simulink model "inverter_spwm_sixty_phases"  (R2024b)
settings: Solver=VariableStepAuto  StartTime=0.0  StopTime=0.1  RelTol=1e-3
libraries: spsMosfetLib x132, spsSeriesRLCBranchLib x65, spsCurrentMeasurementLib x64, spsVoltageMeasurementLib x64, spsTriangleGeneratorLib x20, spsDCVoltageSourceLib x4, spsGroundLib x2, spsThreePhaseSeriesRLCBranchLib x1, sps_lib x1
(part 1 of 2)
settings Model: Creator=Harry  LastModifiedBy=Harry

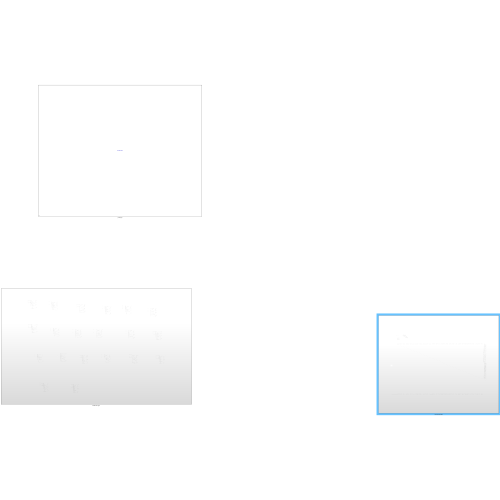
[thumbnail: Simulink's stored preview of the top-level diagram]
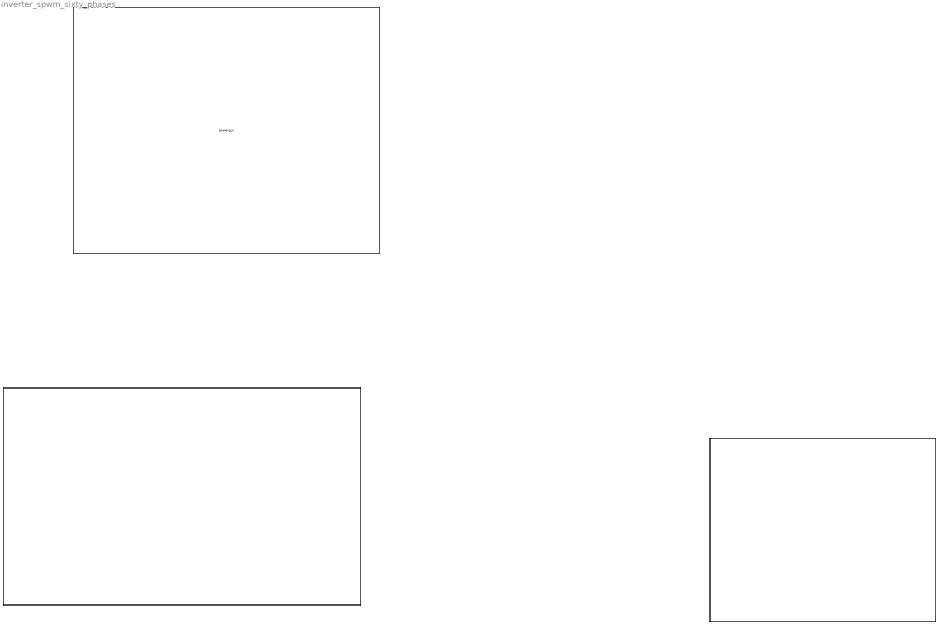
== system inverter_spwm_sixty_phases ==
  Dead time logic : Subsystem
  Inverter switches : Subsystem
  powergui : sps_lib/powergui  Priority=1  SimulationMode=Continuous  SampleTime=50e-6  frequency=60  Iterations=50  frequencyindice=0  Pbase=100e6  ErrMax=1e-4  UnitsV=kV  UnitsW=MW  buscounter=0  FunctionMessages=off  echomessages=off  EnableUseOfTLC=off  CurrentSourceSwitches=off  DisableSnubberDevices=off  DisableRonSwitches=off  DisableVfSwitches=off  DisplayEquations=off  AutomaticDiscreteSolvers=off  SolverType=Tustin/Backward Euler (TBE)  Interpol=off  ExternalGateDelay=off  methode=off  Ts=100  x0status=blocks  SPID=on  SwTol=0  HookPort=off  NonlinearTolerance=1e-4  nMaxIteration=100  ContinueOnMaxIteration=off  RestoreLinks=warning  ResistiveCurrentMeasurement=off  Frange=[0:2:500]  Ylog=off  Xlog=on  ShowGrid=off  save=off  variable=ZData  structure=0  ZoomFFT=off  StartTime=0.0  cycles=1  DisplayStyle=1  fundamental=60  FreqAxis=off  MaxFrequency=1000  frequencyindicesteady=1  RmsSteady=1  display=off

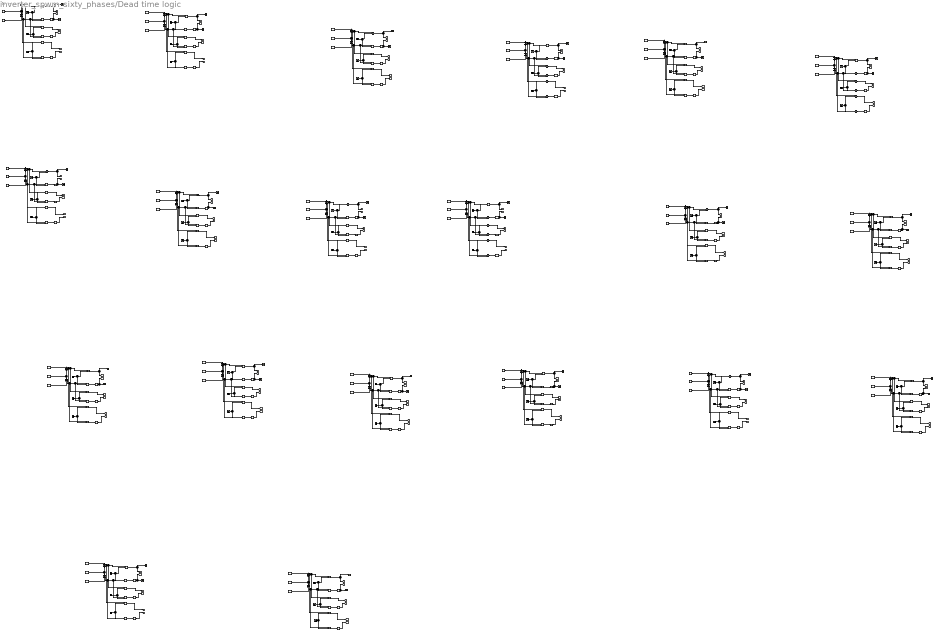
== system inverter_spwm_sixty_phases/Dead time logic ==
  Add{1,3,5,7,9,11,13,15,17,19,21,23,25,27,29,31,33,35,37,39} (20 alike) : Sum
  Add{2,4,6,8,10,12,14,16,18,20,22,24,26,28,30,32,34,36,38,40} (20 alike) : Sum  Inputs=+-
  Constant{1..40} (40 alike) : Constant  Value=0.1
  NOT{1..60} (60 alike) : Logic  Operator=NOT  AllPortsSameDT=off  OutDataTypeStr=boolean
  Relational Operator{,1..119} (120 alike) : RelationalOperator  Operator=<=  OutDataTypeStr=boolean  RndMeth=Simplest  InputSameDT=off
  Scope{,1..39} (40 alike) : Scope
  Sine Wave1 : Sin  Amplitude=0.961  Frequency=2*pi*25  Phase=18*pi/180  SampleTime=0
  Sine Wave10 : Sin  Amplitude=0.961  Frequency=2*pi*25  Phase=54*pi/180  SampleTime=0
  Sine Wave11 : Sin  Amplitude=0.961  Frequency=2*pi*25  Phase=60*pi/180  SampleTime=0
  Sine Wave12 : Sin  Amplitude=0.961  Frequency=2*pi*25  Phase=66*pi/180  SampleTime=0
  Sine Wave13 : Sin  Amplitude=0.961  Frequency=2*pi*25  Phase=72*pi/180  SampleTime=0
  Sine Wave14 : Sin  Amplitude=0.961  Frequency=2*pi*25  Phase=78*pi/180  SampleTime=0
  Sine Wave15 : Sin  Amplitude=0.961  Frequency=2*pi*25  Phase=84*pi/180  SampleTime=0
  Sine Wave16 : Sin  Amplitude=0.961  Frequency=2*pi*25  Phase=90*pi/180  SampleTime=0
  Sine Wave17 : Sin  Amplitude=0.961  Frequency=2*pi*25  Phase=96*pi/180  SampleTime=0
  Sine Wave18 : Sin  Amplitude=0.961  Frequency=2*pi*25  Phase=102*pi/180  SampleTime=0
  Sine Wave19 : Sin  Amplitude=0.961  Frequency=2*pi*25  Phase=324*pi/180  SampleTime=0
  Sine Wave2 : Sin  Amplitude=0.961  Frequency=2*pi*25  Phase=24*pi/180  SampleTime=0
  Sine Wave20 : Sin  Amplitude=0.961  Frequency=2*pi*25  Phase=330*pi/180  SampleTime=0
  Sine Wave21 : Sin  Amplitude=0.961  Frequency=2*pi*25  Phase=336*pi/180  SampleTime=0
  Sine Wave22 : Sin  Amplitude=0.961  Frequency=2*pi*25  Phase=108*pi/180  SampleTime=0
  Sine Wave23 : Sin  Amplitude=0.961  Frequency=2*pi*25  Phase=114*pi/180  SampleTime=0
  Sine Wave24 : Sin  Amplitude=0.961  Frequency=2*pi*25  Phase=120*pi/180  SampleTime=0
  Sine Wave25 : Sin  Amplitude=0.961  Frequency=2*pi*25  Phase=126*pi/180  SampleTime=0
  Sine Wave26 : Sin  Amplitude=0.961  Frequency=2*pi*25  Phase=132*pi/180  SampleTime=0
  Sine Wave27 : Sin  Amplitude=0.961  Frequency=2*pi*25  Phase=138*pi/180  SampleTime=0
  Sine Wave28 : Sin  Amplitude=0.961  Frequency=2*pi*25  Phase=144*pi/180  SampleTime=0
  Sine Wave29 : Sin  Amplitude=0.961  Frequency=2*pi*25  Phase=150*pi/180  SampleTime=0
  Sine Wave3 : Sin  Amplitude=0.961  Frequency=2*pi*25  Phase=30*pi/180  SampleTime=0
  Sine Wave30 : Sin  Amplitude=0.961  Frequency=2*pi*25  Phase=156*pi/180  SampleTime=0
  Sine Wave31 : Sin  Amplitude=0.961  Frequency=2*pi*25  Phase=162*pi/180  SampleTime=0
  Sine Wave32 : Sin  Amplitude=0.961  Frequency=2*pi*25  Phase=168*pi/180  SampleTime=0
  Sine Wave33 : Sin  Amplitude=0.961  Frequency=2*pi*25  Phase=174*pi/180  SampleTime=0
  Sine Wave34 : Sin  Amplitude=0.961  Frequency=2*pi*25  Phase=180*pi/180  SampleTime=0
  Sine Wave35 : Sin  Amplitude=0.961  Frequency=2*pi*25  Phase=186*pi/180  SampleTime=0
  Sine Wave36 : Sin  Amplitude=0.961  Frequency=2*pi*25  Phase=192*pi/180  SampleTime=0
  Sine Wave37 : Sin  Amplitude=0.961  Frequency=2*pi*25  Phase=198*pi/180  SampleTime=0
  Sine Wave38 : Sin  Amplitude=0.961  Frequency=2*pi*25  Phase=204*pi/180  SampleTime=0
  Sine Wave39 : Sin  Amplitude=0.961  Frequency=2*pi*25  Phase=210*pi/180  SampleTime=0
  Sine Wave4 : Sin  Amplitude=0.961  Frequency=2*pi*25  SampleTime=0
  Sine Wave40 : Sin  Amplitude=0.961  Frequency=2*pi*25  Phase=216*pi/180  SampleTime=0
  Sine Wave41 : Sin  Amplitude=0.961  Frequency=2*pi*25  Phase=222*pi/180  SampleTime=0
  Sine Wave42 : Sin  Amplitude=0.961  Frequency=2*pi*25  Phase=228*pi/180  SampleTime=0
  Sine Wave43 : Sin  Amplitude=0.961  Frequency=2*pi*25  Phase=234*pi/180  SampleTime=0
  Sine Wave44 : Sin  Amplitude=0.961  Frequency=2*pi*25  Phase=240*pi/180  SampleTime=0
  Sine Wave45 : Sin  Amplitude=0.961  Frequency=2*pi*25  Phase=246*pi/180  SampleTime=0
  Sine Wave46 : Sin  Amplitude=0.961  Frequency=2*pi*25  Phase=252*pi/180  SampleTime=0
  Sine Wave47 : Sin  Amplitude=0.961  Frequency=2*pi*25  Phase=258*pi/180  SampleTime=0
  Sine Wave48 : Sin  Amplitude=0.961  Frequency=2*pi*25  Phase=264*pi/180  SampleTime=0
  Sine Wave49 : Sin  Amplitude=0.961  Frequency=2*pi*25  Phase=270*pi/180  SampleTime=0
  Sine Wave5 : Sin  Amplitude=0.961  Frequency=2*pi*25  Phase=6*pi/180  SampleTime=0
  Sine Wave50 : Sin  Amplitude=0.961  Frequency=2*pi*25  Phase=276*pi/180  SampleTime=0
  Sine Wave51 : Sin  Amplitude=0.961  Frequency=2*pi*25  Phase=282*pi/180  SampleTime=0
  Sine Wave52 : Sin  Amplitude=0.961  Frequency=2*pi*25  Phase=288*pi/180  SampleTime=0
  Sine Wave53 : Sin  Amplitude=0.961  Frequency=2*pi*25  Phase=294*pi/180  SampleTime=0
  Sine Wave54 : Sin  Amplitude=0.961  Frequency=2*pi*25  Phase=300*pi/180  SampleTime=0
  Sine Wave55 : Sin  Amplitude=0.961  Frequency=2*pi*25  Phase=306*pi/180  SampleTime=0
  Sine Wave56 : Sin  Amplitude=0.961  Frequency=2*pi*25  Phase=312*pi/180  SampleTime=0
  Sine Wave57 : Sin  Amplitude=0.961  Frequency=2*pi*25  Phase=318*pi/180  SampleTime=0
  Sine Wave58 : Sin  Amplitude=0.961  Frequency=2*pi*25  Phase=342*pi/180  SampleTime=0
  Sine Wave59 : Sin  Amplitude=0.961  Frequency=2*pi*25  Phase=348*pi/180  SampleTime=0
  Sine Wave6 : Sin  Amplitude=0.961  Frequency=2*pi*25  Phase=12*pi/180  SampleTime=0
  Sine Wave60 : Sin  Amplitude=0.961  Frequency=2*pi*25  Phase=354*pi/180  SampleTime=0
  Sine Wave7 : Sin  Amplitude=0.961  Frequency=2*pi*25  Phase=36*pi/180  SampleTime=0
  Sine Wave8 : Sin  Amplitude=0.961  Frequency=2*pi*25  Phase=42*pi/180  SampleTime=0
  Sine Wave9 : Sin  Amplitude=0.961  Frequency=2*pi*25  Phase=48*pi/180  SampleTime=0
  Triangle Generator{,1..19} (20 alike) : spsTriangleGeneratorLib/Triangle Generator  Freq=2000  Phase=90  Ts=0
  tag scope: s100=global, s101=global, s102=global, s103=global, s104=global, s105=global, s106=global, s107=global, s108=global, s109=global, s10=global, s110=global, s111=global, s112=global, s113=global, s114=global, s115=global, s116=global, s117=global, s118=global, s119=global, s11=global, s120=global, s12=global, s13=global, s14=global, s15=global, s16=global, s17=global, s18=global, s19=global, s1=global, s20=global, s21=global, s22=global, s23=global, s24=global, s25=global, s26=global, s27=global, s28=global, s29=global, s2=global, s30=global, s31=global, s32=global, s33=global, s34=global, s35=global, s36=global, s37=global, s38=global, s39=global, s3=global, s40=global, s41=global, s42=global, s43=global, s44=global, s45=global, s46=global, s47=global, s48=global, s49=global, s4=global, s50=global, s51=global, s52=global, s53=global, s54=global, s55=global, s56=global, s57=global, s58=global, s59=global, s5=global, s60=global, s61=global, s62=global, s63=global, s64=global, s65=global, s66=global, s67=global, s68=global, s69=global, s6=global, s70=global, s71=global, s72=global, s73=global, s74=global, s75=global, s76=global, s77=global, s78=global, s79=global, s7=global, s80=global, s81=global, s82=global, s83=global, s84=global, s85=global, s86=global, s87=global, s88=global, s89=global, s8=global, s90=global, s91=global, s92=global, s93=global, s94=global, s95=global, s96=global, s97=global, s98=global, s99=global, s9=global
  wires:
  Relational Operator5/1 -> NOT5/1
  Add8/1 -> Relational Operator4/1, Relational Operator5/1, Relational Operator1/1
  Relational Operator3/1 -> [s5]
  Sine Wave4/1 -> Relational Operator/2, Relational Operator1/2
  Sine Wave6/1 -> Relational Operator4/2, Relational Operator3/2
  Relational Operator2/1 -> [s3]
  Sine Wave5/1 -> Relational Operator5/2, Relational Operator2/2
  Relational Operator4/1 -> NOT6/1
  Triangle Generator/1 -> Add8/1, Add7/2
  NOT5/1 -> [s4]
  Relational Operator1/1 -> NOT4/1
  NOT6/1 -> [s6]
  Constant2/1 -> Add7/1
  Relational Operator/1 -> [s1], Scope1/1
  Constant3/1 -> Add8/2
  NOT4/1 -> [s2], Scope/1
  Add7/1 -> Relational Operator3/1, Relational Operator2/1, Relational Operator/1
  NOT24/1 -> [s42]
  Triangle Generator7/1 -> Add16/1, Add15/2
  Sine Wave23/1 -> Relational Operator47/2, Relational Operator44/2
  Sine Wave22/1 -> Relational Operator42/2, Relational Operator43/2
  Relational Operator44/1 -> [s39]
  Relational Operator43/1 -> NOT22/1
  Sine Wave24/1 -> Relational Operator46/2, Relational Operator45/2
  Relational Operator45/1 -> [s41]
  Relational Operator47/1 -> NOT23/1
  Add16/1 -> Relational Operator46/1, Relational Operator47/1, Relational Operator43/1
  Relational Operator46/1 -> NOT24/1
  Constant16/1 -> Add16/2
  NOT22/1 -> [s38], Scope14/1
  Relational Operator42/1 -> [s37], Scope15/1
  Constant15/1 -> Add15/1
  Add15/1 -> Relational Operator45/1, Relational Operator44/1, Relational Operator42/1
  NOT23/1 -> [s40]
  NOT27/1 -> [s48]
  Triangle Generator8/1 -> Add18/1, Add17/2
  Sine Wave26/1 -> Relational Operator53/2, Relational Operator50/2
  Sine Wave25/1 -> Relational Operator48/2, Relational Operator49/2
  Relational Operator50/1 -> [s45]
  Relational Operator49/1 -> NOT25/1
  Sine Wave27/1 -> Relational Operator52/2, Relational Operator51/2
  Relational Operator51/1 -> [s47]
  Relational Operator53/1 -> NOT26/1
  Add18/1 -> Relational Operator52/1, Relational Operator53/1, Relational Operator49/1
  Relational Operator52/1 -> NOT27/1
  Constant18/1 -> Add18/2
  NOT25/1 -> [s44], Scope16/1
  Relational Operator48/1 -> [s43], Scope17/1
  Constant17/1 -> Add17/1
  Add17/1 -> Relational Operator51/1, Relational Operator50/1, Relational Operator48/1
  NOT26/1 -> [s46]
  NOT30/1 -> [s54]
  Triangle Generator9/1 -> Add20/1, Add19/2
  Sine Wave29/1 -> Relational Operator59/2, Relational Operator56/2
  Sine Wave28/1 -> Relational Operator54/2, Relational Operator55/2
  Relational Operator56/1 -> [s51]
  Relational Operator55/1 -> NOT28/1
  Sine Wave30/1 -> Relational Operator58/2, Relational Operator57/2
  Relational Operator57/1 -> [s53]
  Relational Operator59/1 -> NOT29/1
  Add20/1 -> Relational Operator58/1, Relational Operator59/1, Relational Operator55/1
  Relational Operator58/1 -> NOT30/1
  Constant20/1 -> Add20/2
  NOT28/1 -> [s50], Scope18/1
  Relational Operator54/1 -> [s49], Scope19/1
  Constant19/1 -> Add19/1
  Add19/1 -> Relational Operator57/1, Relational Operator56/1, Relational Operator54/1
  NOT29/1 -> [s52]
  NOT33/1 -> [s60]
  Triangle Generator10/1 -> Add22/1, Add21/2
  Sine Wave32/1 -> Relational Operator65/2, Relational Operator62/2
  Sine Wave31/1 -> Relational Operator60/2, Relational Operator61/2
  Relational Operator62/1 -> [s57]
  Relational Operator61/1 -> NOT31/1
  Sine Wave33/1 -> Relational Operator64/2, Relational Operator63/2
  Relational Operator63/1 -> [s59]
  Relational Operator65/1 -> NOT32/1
  Add22/1 -> Relational Operator64/1, Relational Operator65/1, Relational Operator61/1
  Relational Operator64/1 -> NOT33/1
  Constant22/1 -> Add22/2
  NOT31/1 -> [s56], Scope20/1
  Relational Operator60/1 -> [s55], Scope21/1
  Constant21/1 -> Add21/1
  Add21/1 -> Relational Operator63/1, Relational Operator62/1, Relational Operator60/1
  NOT32/1 -> [s58]
  NOT36/1 -> [s66]
  Triangle Generator11/1 -> Add24/1, Add23/2
  Sine Wave35/1 -> Relational Operator71/2, Relational Operator68/2
  Sine Wave34/1 -> Relational Operator66/2, Relational Operator67/2
  Relational Operator68/1 -> [s63]
  Relational Operator67/1 -> NOT34/1
  Sine Wave36/1 -> Relational Operator70/2, Relational Operator69/2
  Relational Operator69/1 -> [s65]
  Relational Operator71/1 -> NOT35/1
  Add24/1 -> Relational Operator70/1, Relational Operator71/1, Relational Operator67/1
  Relational Operator70/1 -> NOT36/1
  Constant24/1 -> Add24/2
  NOT34/1 -> [s62], Scope22/1
  Relational Operator66/1 -> [s61], Scope23/1
  Constant23/1 -> Add23/1
  Add23/1 -> Relational Operator69/1, Relational Operator68/1, Relational Operator66/1
  NOT35/1 -> [s64]
  NOT39/1 -> [s72]
  Triangle Generator12/1 -> Add26/1, Add25/2
  Sine Wave38/1 -> Relational Operator77/2, Relational Operator74/2
  Sine Wave37/1 -> Relational Operator72/2, Relational Operator73/2
  Relational Operator74/1 -> [s69]
  Relational Operator73/1 -> NOT37/1
  Sine Wave39/1 -> Relational Operator76/2, Relational Operator75/2
  Relational Operator75/1 -> [s71]
  Relational Operator77/1 -> NOT38/1
  Add26/1 -> Relational Operator76/1, Relational Operator77/1, Relational Operator73/1
  Relational Operator76/1 -> NOT39/1
  Constant26/1 -> Add26/2
  NOT37/1 -> [s68], Scope24/1
  Relational Operator72/1 -> [s67], Scope25/1
  Constant25/1 -> Add25/1
  Add25/1 -> Relational Operator75/1, Relational Operator74/1, Relational Operator72/1
  NOT38/1 -> [s70]
  NOT42/1 -> [s78]
  Triangle Generator13/1 -> Add28/1, Add27/2
  Sine Wave41/1 -> Relational Operator83/2, Relational Operator80/2
  Sine Wave40/1 -> Relational Operator78/2, Relational Operator79/2
  Relational Operator80/1 -> [s75]
  Relational Operator79/1 -> NOT40/1
  Sine Wave42/1 -> Relational Operator82/2, Relational Operator81/2
  Relational Operator81/1 -> [s77]
  Relational Operator83/1 -> NOT41/1
  Add28/1 -> Relational Operator82/1, Relational Operator83/1, Relational Operator79/1
  Relational Operator82/1 -> NOT42/1
  Constant28/1 -> Add28/2
  NOT40/1 -> [s74], Scope26/1
  Relational Operator78/1 -> [s73], Scope27/1
  Constant27/1 -> Add27/1
  Add27/1 -> Relational Operator81/1, Relational Operator80/1, Relational Operator78/1
  NOT41/1 -> [s76]
  NOT45/1 -> [s84]
  Triangle Generator14/1 -> Add30/1, Add29/2
  Sine Wave44/1 -> Relational Operator89/2, Relational Operator86/2
  Sine Wave43/1 -> Relational Operator84/2, Relational Operator85/2
  Relational Operator86/1 -> [s81]
  Relational Operator85/1 -> NOT43/1
  Sine Wave45/1 -> Relational Operator88/2, Relational Operator87/2
  Relational Operator87/1 -> [s83]
  Relational Operator89/1 -> NOT44/1
  Add30/1 -> Relational Operator88/1, Relational Operator89/1, Relational Operator85/1
  Relational Operator88/1 -> NOT45/1
  Constant30/1 -> Add30/2
  NOT43/1 -> [s80], Scope28/1
  Relational Operator84/1 -> [s79], Scope29/1
  Constant29/1 -> Add29/1
  Add29/1 -> Relational Operator87/1, Relational Operator86/1, Relational Operator84/1
  NOT44/1 -> [s82]
  NOT48/1 -> [s90]
  Triangle Generator15/1 -> Add32/1, Add31/2
  Sine Wave47/1 -> Relational Operator95/2, Relational Operator92/2
  Sine Wave46/1 -> Relational Operator90/2, Relational Operator91/2
  Relational Operator92/1 -> [s87]
  Relational Operator91/1 -> NOT46/1
  Sine Wave48/1 -> Relational Operator94/2, Relational Operator93/2
  Relational Operator93/1 -> [s89]
  Relational Operator95/1 -> NOT47/1
  Add32/1 -> Relational Operator94/1, Relational Operator95/1, Relational Operator91/1
  Relational Operator94/1 -> NOT48/1
  Constant32/1 -> Add32/2
  NOT46/1 -> [s86], Scope30/1
  Relational Operator90/1 -> [s85], Scope31/1
  Constant31/1 -> Add31/1
  Add31/1 -> Relational Operator93/1, Relational Operator92/1, Relational Operator90/1
  NOT47/1 -> [s88]
  NOT51/1 -> [s96]
  Triangle Generator16/1 -> Add34/1, Add33/2
  Sine Wave50/1 -> Relational Operator101/2, Relational Operator98/2
  Sine Wave49/1 -> Relational Operator96/2, Relational Operator97/2
  Relational Operator98/1 -> [s93]
  Relational Operator97/1 -> NOT49/1
  Sine Wave51/1 -> Relational Operator100/2, Relational Operator99/2
  Relational Operator99/1 -> [s95]
  Relational Operator101/1 -> NOT50/1
  Add34/1 -> Relational Operator100/1, Relational Operator101/1, Relational Operator97/1
  Relational Operator100/1 -> NOT51/1
  Constant34/1 -> Add34/2
  NOT49/1 -> [s92], Scope32/1
  Relational Operator96/1 -> [s91], Scope33/1
  Constant33/1 -> Add33/1
  Add33/1 -> Relational Operator99/1, Relational Operator98/1, Relational Operator96/1
  NOT50/1 -> [s94]
  NOT54/1 -> [s102]
  Triangle Generator17/1 -> Add36/1, Add35/2
  Sine Wave53/1 -> Relational Operator107/2, Relational Operator104/2
  Sine Wave52/1 -> Relational Operator102/2, Relational Operator103/2
  Relational Operator104/1 -> [s99]
  Relational Operator103/1 -> NOT52/1
  Sine Wave54/1 -> Relational Operator106/2, Relational Operator105/2
  Relational Operator105/1 -> [s101]
  Relational Operator107/1 -> NOT53/1
  Add36/1 -> Relational Operator106/1, Relational Operator107/1, Relational Operator103/1
  Relational Operator106/1 -> NOT54/1
  Constant36/1 -> Add36/2
  NOT52/1 -> [s98], Scope34/1
  Relational Operator102/1 -> [s97], Scope35/1
  Constant35/1 -> Add35/1
  Add35/1 -> Relational Operator105/1, Relational Operator104/1, Relational Operator102/1
  NOT53/1 -> [s100]
  NOT57/1 -> [s108]
  Triangle Generator18/1 -> Add38/1, Add37/2
  Sine Wave56/1 -> Relational Operator113/2, Relational Operator110/2
  Sine Wave55/1 -> Relational Operator108/2, Relational Operator109/2
  Relational Operator110/1 -> [s105]
  Relational Operator109/1 -> NOT55/1
  Sine Wave57/1 -> Relational Operator112/2, Relational Operator111/2
  Relational Operator111/1 -> [s107]
  Relational Operator113/1 -> NOT56/1
  Add38/1 -> Relational Operator112/1, Relational Operator113/1, Relational Operator109/1
  Relational Operator112/1 -> NOT57/1
  Constant38/1 -> Add38/2
  NOT55/1 -> [s104], Scope36/1
  Relational Operator108/1 -> [s103], Scope37/1
  Constant37/1 -> Add37/1
  Add37/1 -> Relational Operator111/1, Relational Operator110/1, Relational Operator108/1
  NOT56/1 -> [s106]
  NOT3/1 -> [s12]
  Triangle Generator1/1 -> Add2/1, Add1/2
  Sine Wave2/1 -> Relational Operator11/2, Relational Operator8/2
  Sine Wave1/1 -> Relational Operator6/2, Relational Operator7/2
  Relational Operator8/1 -> [s9]
  Relational Operator7/1 -> NOT1/1
  Sine Wave3/1 -> Relational Operator10/2, Relational Operator9/2
  Relational Operator9/1 -> [s11]
  Relational Operator11/1 -> NOT2/1
  Add2/1 -> Relational Operator10/1, Relational Operator11/1, Relational Operator7/1
  Relational Operator10/1 -> NOT3/1
  Constant4/1 -> Add2/2
  NOT1/1 -> [s8], Scope2/1
  Relational Operator6/1 -> [s7], Scope3/1
  Constant1/1 -> Add1/1
  Add1/1 -> Relational Operator9/1, Relational Operator8/1, Relational Operator6/1
  NOT2/1 -> [s10]
  NOT9/1 -> [s18]
  Triangle Generator2/1 -> Add4/1, Add3/2
  Sine Wave8/1 -> Relational Operator17/2, Relational Operator14/2
  Sine Wave7/1 -> Relational Operator12/2, Relational Operator13/2
  Relational Operator14/1 -> [s15]
  Relational Operator13/1 -> NOT7/1
  Sine Wave9/1 -> Relational Operator16/2, Relational Operator15/2
  Relational Operator15/1 -> [s17]
  Relational Operator17/1 -> NOT8/1
  Add4/1 -> Relational Operator16/1, Relational Operator17/1, Relational Operator13/1
  Relational Operator16/1 -> NOT9/1
  Constant6/1 -> Add4/2
  NOT7/1 -> [s14], Scope4/1
  Relational Operator12/1 -> [s13], Scope5/1
  Constant5/1 -> Add3/1
  Add3/1 -> Relational Operator15/1, Relational Operator14/1, Relational Operator12/1
  NOT8/1 -> [s16]
  NOT12/1 -> [s24]
  Triangle Generator3/1 -> Add6/1, Add5/2
  Sine Wave11/1 -> Relational Operator23/2, Relational Operator20/2
  Sine Wave10/1 -> Relational Operator18/2, Relational Operator19/2
  Relational Operator20/1 -> [s21]
  Relational Operator19/1 -> NOT10/1
  Sine Wave12/1 -> Relational Operator22/2, Relational Operator21/2
  Relational Operator21/1 -> [s23]
  Relational Operator23/1 -> NOT11/1
  Add6/1 -> Relational Operator22/1, Relational Operator23/1, Relational Operator19/1
  Relational Operator22/1 -> NOT12/1
  Constant8/1 -> Add6/2
  NOT10/1 -> [s20], Scope6/1
  Relational Operator18/1 -> [s19], Scope7/1
  Constant7/1 -> Add5/1
  Add5/1 -> Relational Operator21/1, Relational Operator20/1, Relational Operator18/1
  NOT11/1 -> [s22]
  NOT15/1 -> [s30]
  Triangle Generator4/1 -> Add10/1, Add9/2
  Sine Wave14/1 -> Relational Operator29/2, Relational Operator26/2
  Sine Wave13/1 -> Relational Operator24/2, Relational Operator25/2
  Relational Operator26/1 -> [s27]
  Relational Operator25/1 -> NOT13/1
  Sine Wave15/1 -> Relational Operator28/2, Relational Operator27/2
  Relational Operator27/1 -> [s29]
  Relational Operator29/1 -> NOT14/1
  Add10/1 -> Relational Operator28/1, Relational Operator29/1, Relational Operator25/1
  Relational Operator28/1 -> NOT15/1
  Constant10/1 -> Add10/2
  NOT13/1 -> [s26], Scope8/1
  Relational Operator24/1 -> [s25], Scope9/1
  Constant9/1 -> Add9/1
  Add9/1 -> Relational Operator27/1, Relational Operator26/1, Relational Operator24/1
  NOT14/1 -> [s28]
  NOT18/1 -> [s36]
  Triangle Generator5/1 -> Add12/1, Add11/2
  Sine Wave17/1 -> Relational Operator35/2, Relational Operator32/2
  Sine Wave16/1 -> Relational Operator30/2, Relational Operator31/2
  Relational Operator32/1 -> [s33]
  Relational Operator31/1 -> NOT16/1
  Sine Wave18/1 -> Relational Operator34/2, Relational Operator33/2
  Relational Operator33/1 -> [s35]
  Relational Operator35/1 -> NOT17/1
  Add12/1 -> Relational Operator34/1, Relational Operator35/1, Relational Operator31/1
  Relational Operator34/1 -> NOT18/1
  Constant12/1 -> Add12/2
  NOT16/1 -> [s32], Scope10/1
  Relational Operator30/1 -> [s31], Scope11/1
  Constant11/1 -> Add11/1
  Add11/1 -> Relational Operator33/1, Relational Operator32/1, Relational Operator30/1
  NOT17/1 -> [s34]
  NOT21/1 -> [s114]
  Triangle Generator6/1 -> Add14/1, Add13/2
  Sine Wave20/1 -> Relational Operator41/2, Relational Operator38/2
  Sine Wave19/1 -> Relational Operator36/2, Relational Operator37/2
  Relational Operator38/1 -> [s111]
  Relational Operator37/1 -> NOT19/1
  Sine Wave21/1 -> Relational Operator40/2, Relational Operator39/2
  Relational Operator39/1 -> [s113]
  Relational Operator41/1 -> NOT20/1
  Add14/1 -> Relational Operator40/1, Relational Operator41/1, Relational Operator37/1
  Relational Operator40/1 -> NOT21/1
  Constant14/1 -> Add14/2
  NOT19/1 -> [s110], Scope12/1
  Relational Operator36/1 -> [s109], Scope13/1
  Constant13/1 -> Add13/1
  Add13/1 -> Relational Operator39/1, Relational Operator38/1, Relational Operator36/1
  NOT20/1 -> [s112]
  NOT60/1 -> [s120]
  Triangle Generator19/1 -> Add40/1, Add39/2
  Sine Wave59/1 -> Relational Operator119/2, Relational Operator116/2
  Sine Wave58/1 -> Relational Operator114/2, Relational Operator115/2
  Relational Operator116/1 -> [s117]
  Relational Operator115/1 -> NOT58/1
  Sine Wave60/1 -> Relational Operator118/2, Relational Operator117/2
  Relational Operator117/1 -> [s119]
  Relational Operator119/1 -> NOT59/1
  Add40/1 -> Relational Operator118/1, Relational Operator119/1, Relational Operator115/1
  Relational Operator118/1 -> NOT60/1
  Constant40/1 -> Add40/2
  NOT58/1 -> [s116], Scope38/1
  Relational Operator114/1 -> [s115], Scope39/1
  Constant39/1 -> Add39/1
  Add39/1 -> Relational Operator117/1, Relational Operator116/1, Relational Operator114/1
  NOT59/1 -> [s118]
